simulink model "px4demo_Serial_TxRxtest"  (R2016b)
settings: Solver=FixedStepDiscrete  StartTime=0.0  StopTime=inf  FixedStep=0.01  RelTol=1e-3  EnableMultiTasking=on
libraries: pixhawk_slib_ADC_serial x2, pixhawk_slib_uORB_RW x2
settings Model: Creator=darenlee  LastModifiedBy=E6320
settings DataIOCC: LimitDataPoints=on  SaveFormat=StructureWithTime
settings OptimizationCC: DefaultParameterBehavior=Inlined  LifeSpan=1  MaxStackSize=64
settings DebuggingCC: AllowSymbolicDim=off  SFUnexpectedBacktrackingDiag=warning  SFNoUnconditionalDefaultTransitionDiag=warning  SFExecutionAtInitializationDiag=none
settings HardwareCC: ProdBitPerPointer=32  ProdBitPerSizeT=32  ProdBitPerPtrDiffT=32  ProdLargestAtomicInteger=Long  ProdLargestAtomicFloat=Double  ProdIntDivRoundTo=Undefined  ProdWordSize=32  ProdHWDeviceType=ARM Compatible->ARM Cortex
settings ModelReferenceCC: PropagateSignalLabelsOutOfModel=off
settings RTWCC: SystemTargetFile=ert.tlc  HardwareBoard=Pixhawk PX4  TLCOptions=-aInlineSetEventsForThisBaseRateFcn=TLC_FALSE -aSuppressMultiTaskScheduler=TLC_FALSE -aRateBasedStepFcn=0  TemplateMakefile=ert_default_tmf  Description=Embedded Coder  GenerateReport=on  Toolchain=Pixhawk Toolchain  IncludeHyperlinkInReport=on  LaunchReport=on  GenerateTraceInfo=on  GenerateTraceReport=on  GenerateTraceReportSl=on  GenerateTraceReportSf=on  GenerateTraceReportEml=on
settings CodeAppCC: IgnoreCustomStorageClasses=off
settings ERTTargetCC: ExtModeTransport=1  ExtModeMexFile=ext_serial_win32_comm  ExtModeMexArgs=1 8 115200  ERTCustomFileTemplate=PX4_codertarget_file_process.tlc  ConvertIfToSwitch=off  SuppressUnreachableDefaultCases=off
settings ConfigComp: CovMetricSettings=dw  CovHtmlReporting=on  CovSaveCumulativeToWorkspaceVar=on  CovSaveSingleToWorkspaceVar=on  CovExternalEMLEnable=off

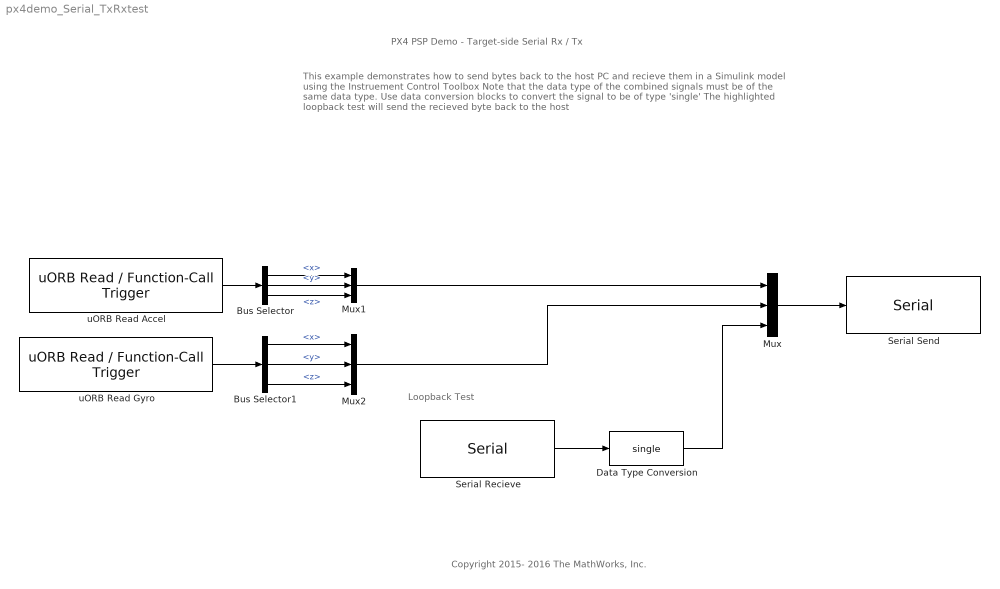
== system px4demo_Serial_TxRxtest ==
  note: Loopback Test
  note: This example demonstrates how to send bytes back to the host PC
      | and recieve them in a Simulink model using the Instruement Control Toolbox
      |
      | Note that the data type of the combined signals must be of the same data type.
      | Use data conversion blocks to convert the signal to be of type 'single'
      |
      | The highlighted loopback test will send the recieved byte back to the host
  note: PX4 PSP Demo - Target-side Serial Rx / Tx
  note: Copyright 2015- 2016 The MathWorks, Inc.
  Bus Selector : BusSelector  OutputSignals=x,y,z
  Bus Selector1 : BusSelector  OutputSignals=x,y,z
  Data Type Conversion : DataTypeConversion  OutDataTypeStr=single
  Mux : Mux  Inputs=3
  Mux1 : Mux  Inputs=3
  Mux2 : Mux  Inputs=3
  Serial Recieve : pixhawk_slib_ADC_serial/Serial  DeviceName=/dev/ttyACM0  ReadOrWrite=Reading  BaudRateStr=115200  block=off  WriteStatus=off  Terminator=off  Header=off  NumBytesRead=1  TerminatorChar=\n  HeaderData=[ uint8( hex2dec( 'DE' ) ), uint8( hex2dec( 'AD' ) ), uint8( hex2dec( 'C0' ) ), uint8( hex2dec( 'DE' ) ) ]  SimulateUsing=Code generation
  Serial Send : pixhawk_slib_ADC_serial/Serial  DeviceName=/dev/ttyACM0  ReadOrWrite=Writing  BaudRateStr=115200  block=off  WriteStatus=on  Terminator=off  Header=off  NumBytesRead=4  TerminatorChar=\n  HeaderData=[ uint8( hex2dec( 'DE' ) ), uint8( hex2dec( 'AD' ) ), uint8( hex2dec( 'C0' ) ), uint8( hex2dec( 'DE' ) ) ]  SimulateUsing=Code generation
  uORB Read Accel : pixhawk_slib_uORB_RW/uORB Read // Function-Call Trigger  uORB_Topic_str='sensor_accel'  BusObjVar=Bus: sensor_accel_SL  uORB_Interval=20  AsyncOutput=off  Fcn_call_select=Generate Function Call Signal  TaskName='Task0'  Poll_timeout=100  Ts=-1
  uORB Read Gyro : pixhawk_slib_uORB_RW/uORB Read // Function-Call Trigger  uORB_Topic_str='sensor_gyro'  BusObjVar=Bus: sensor_gyro_SL  uORB_Interval=20  AsyncOutput=off  Fcn_call_select=Generate Function Call Signal  TaskName='Task0'  Poll_timeout=100  Ts=-1
  wires:
  Mux/1 -> Serial Send/1
  Serial Recieve/1 -> Data Type Conversion/1
  Data Type Conversion/1 -> Mux/3
  uORB Read Accel/1 -> Bus Selector/1
  Bus Selector/1 -> Mux1/1  "<x>"
  Bus Selector/2 -> Mux1/2  "<y>"
  Bus Selector/3 -> Mux1/3  "<z>"
  Mux1/1 -> Mux/1
  Mux2/1 -> Mux/2
  uORB Read Gyro/1 -> Bus Selector1/1
  Bus Selector1/2 -> Mux2/2  "<y>"
  Bus Selector1/1 -> Mux2/1  "<x>"
  Bus Selector1/3 -> Mux2/3  "<z>"
